simulink model "valveModel"  (R2018a)
settings: Solver=VariableStepAuto  StartTime=0.0  StopTime=1  RelTol=1e-3
settings Model: Creator=Ruben  LastModifiedBy=Ruben

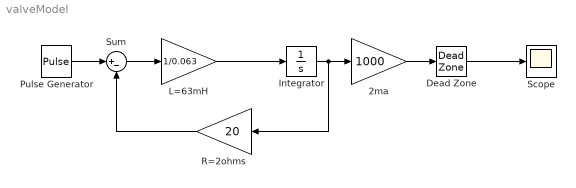
== system valveModel ==
  2ma : Gain  Gain=1000
  Dead Zone : DeadZone  LowerValue=0  UpperValue=250  SaturateOnIntegerOverflow=on
  Integrator : Integrator
  L=63mH : Gain  Gain=1/0.063
  Pulse Generator : DiscretePulseGenerator  PulseType=Time based  Amplitude=12  Period=10  PulseWidth=5
  R=2ohms : Gain  Gain=20
  Scope : Scope
  Sum : Sum  Inputs=|+-
  wires:
  Sum/1 -> L=63mH/1
  L=63mH/1 -> Integrator/1
  R=2ohms/1 -> Sum/2
  Pulse Generator/1 -> Sum/1
  Dead Zone/1 -> Scope/1
  2ma/1 -> Dead Zone/1
  Integrator/1 -> R=2ohms/1, 2ma/1
